simulink model "MatlabSimulink"  (R2021a)
settings: Solver=VariableStepAuto  StartTime=0.0  StopTime=10.0  RelTol=1e-3
undefined symbols (not defined in the file or in its folder): B, Mp, v0, x0
settings Model: Creator=schmi  LastModifiedBy=schmi

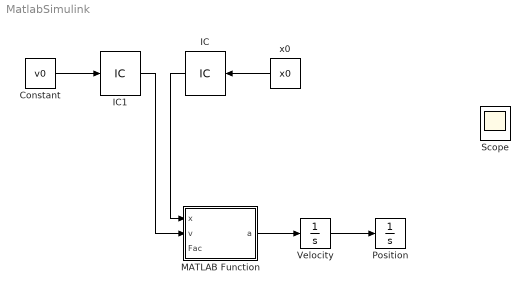
== system MatlabSimulink ==
  Constant : Constant  Value=v0
  IC : InitialCondition
  IC1 : InitialCondition
  MATLAB Function : MATLAB Function  TreatAsAtomicUnit=on
  Position : Integrator
  Scope : Scope  NumInputPorts=3
  Velocity : Integrator
  x0 : Constant  Value=x0
  wires:
  MATLAB Function/1(a) -> Velocity/1
  IC/1 -> MATLAB Function/1(x)
  Constant/1 -> IC1/1
  x0/1 -> IC/1
  Velocity/1 -> Position/1
  IC1/1 -> MATLAB Function/2(v)

== matlab function MatlabSimulink/MATLAB Function ==
  data: x input; a output; v input; Mp parameter; B parameter; Fac input
function a = fcn(x, v, Mp, B, Fac)

a = 1/Mp * (Fac - B*v);
